simulink model "Lab05S"  (R2023b)
settings: Solver=VariableStepAuto  StartTime=0.0  StopTime=10.0  RelTol=1e-3
values from neighbouring files (symbols this model uses):
  A = [0 -1 5; 0 0 3; 0 0 -2]    [Lab01.m]    (also in Lab03.m = double(subs(A,x,x_eq)); Lab04.m = double(subs(A,[x u],[x_eq u_eq])); Lab05.m = [0 1; -3 -4])
  alpha = inv(-C*((A-B*K)\B))    [Lab04.m]    (also in Lab05.m; Prob1.m = 0.05; Prob2.m = 0.05; Prob3.m = 0.05)
  alpha_4 = inv(-C*((A-B*K_4)\B))    [Lab05.m]
  B = [1 1 1]'    [Lab01.m]    (also in Lab03.m = double(subs(B,u,u_eq)); Lab04.m = double(subs(B,[x u],[x_eq u_eq])); Lab05.m = [0 ; 1])
  B_reale = B.*epsilon    [Lab05.m]
  C = [0 0 5]    [Lab01.m]    (also in Lab03.m = double(subs(C,x,x_eq)); Lab04.m = double(subs(C,x,x_eq)); Lab05.m = [2 1])
  D = double(subs(D,u,u_eq))    [Lab03.m]    (also in Lab04.m; Lab05.m = 0)
  K = place(A,B,lambda_k)    [Lab04.m]    (also in Lab05.m)
  K_4 = place(A,B,lambda_k_4)    [Lab05.m]
  L = place(A',C',lambda_o)'    [Lab04.m]    (also in Lab05.m; Prob1.m = -Kc*Gp*Ga; Prob2.m = -Kc*Gp*Ga; Prob3.m = -Kc*Gp*Ga)
  L_6 = place(A',C',lambda_o_6)'    [Lab05.m]
  L_7 = place(A',C',lambda_o_7)'    [Lab05.m]
settings Model: Creator=matteo  LastModifiedBy=matteo

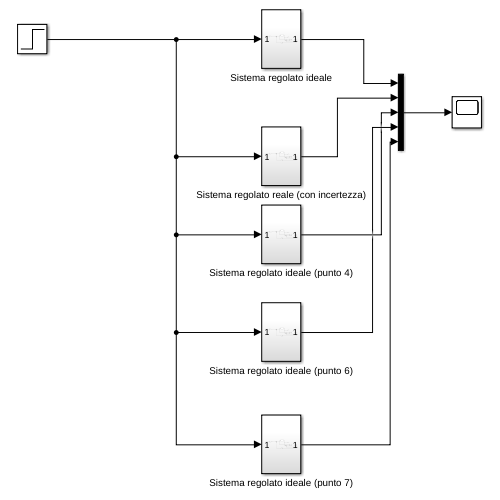
[thumbnail: Simulink's stored preview of the top-level diagram]
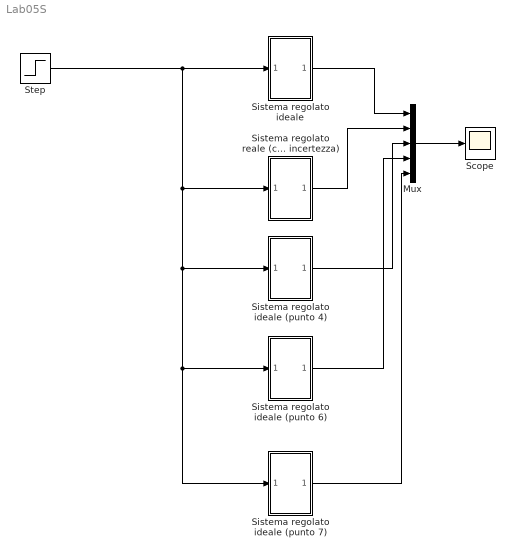
== system Lab05S ==
  Mux : Mux  Inputs=5
  Scope : Scope
  Sistema regolato ideale : Subsystem
  Sistema regolato ideale (punto 4) : Subsystem
  Sistema regolato ideale (punto 6) : Subsystem
  Sistema regolato ideale (punto 7) : Subsystem
  Sistema regolato reale (con incertezza) : Subsystem
  Step : Step  Time=0  SampleTime=0
  wires:
  Step/1 -> Sistema regolato ideale/1(In1), Sistema regolato reale (con incertezza)/1(In1), Sistema regolato ideale (punto 4)/1(In1), Sistema regolato ideale (punto 6)/1(In1), Sistema regolato ideale (punto 7)/1(In1)
  Sistema regolato ideale/1(Out1) -> Mux/1
  Mux/1 -> Scope/1
  Sistema regolato ideale (punto 4)/1(Out1) -> Mux/3
  Sistema regolato ideale (punto 6)/1(Out1) -> Mux/4
  Sistema regolato ideale (punto 7)/1(Out1) -> Mux/5
  Sistema regolato reale (con incertezza)/1(Out1) -> Mux/2

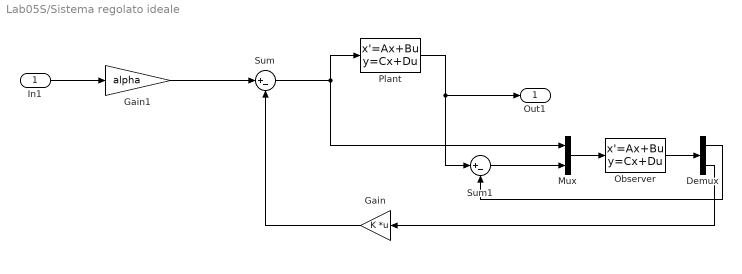
== system Lab05S/Sistema regolato ideale ==
  In1 : Inport
  Demux : Demux  Outputs=2
  Gain : Gain  Gain=K  Multiplication=Matrix(K*u)
  Gain1 : Gain  Gain=alpha
  Mux : Mux  Inputs=2
  Observer : StateSpace  A=A  B=[B L]  C=[C; eye(2)]  D=zeros(3,2)  InitialCondition=0
  Plant : StateSpace  A=A  B=B  C=C  D=D  InitialCondition=[0 0]'
  Sum : Sum  Inputs=|+-
  Sum1 : Sum  Inputs=|+-
  Out1 : Outport
  wires:
  Sum1/1 -> Mux/2
  In1/1 -> Gain1/1
  Gain/1 -> Sum/2
  Demux/1 -> Sum1/2
  Mux/1 -> Observer/1
  Observer/1 -> Demux/1
  Gain1/1 -> Sum/1
  Demux/2 -> Gain/1
  Sum/1 -> Mux/1, Plant/1
  Plant/1 -> Out1/1, Sum1/1

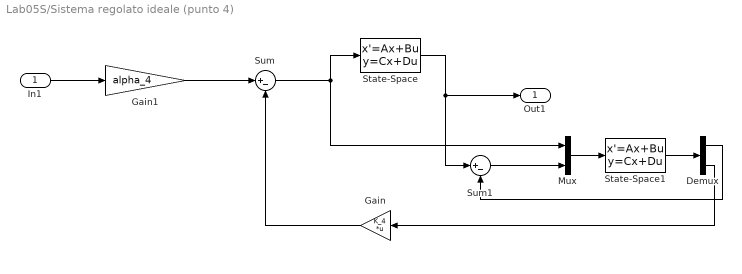
== system Lab05S/Sistema regolato ideale (punto 4) ==
  In1 : Inport
  Demux : Demux  Outputs=2
  Gain : Gain  Gain=K_4  Multiplication=Matrix(K*u)
  Gain1 : Gain  Gain=alpha_4
  Mux : Mux  Inputs=2
  State-Space : StateSpace  A=A  B=B  C=C  D=D  InitialCondition=[0 0]'
  State-Space1 : StateSpace  A=A  B=[B L]  C=[C; eye(2)]  D=zeros(3,2)  InitialCondition=0
  Sum : Sum  Inputs=|+-
  Sum1 : Sum  Inputs=|+-
  Out1 : Outport
  wires:
  Sum1/1 -> Mux/2
  In1/1 -> Gain1/1
  Gain/1 -> Sum/2
  Demux/1 -> Sum1/2
  Mux/1 -> State-Space1/1
  State-Space1/1 -> Demux/1
  Gain1/1 -> Sum/1
  Demux/2 -> Gain/1
  Sum/1 -> Mux/1, State-Space/1
  State-Space/1 -> Out1/1, Sum1/1

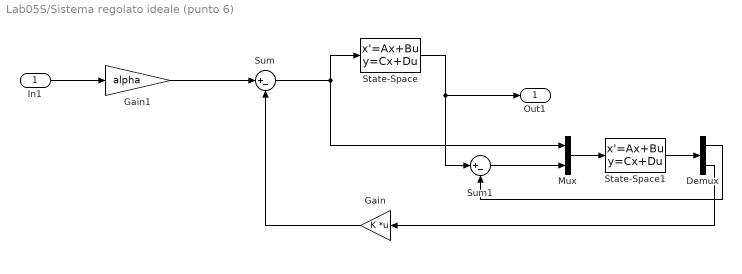
== system Lab05S/Sistema regolato ideale (punto 6) ==
  In1 : Inport
  Demux : Demux  Outputs=2
  Gain : Gain  Gain=K  Multiplication=Matrix(K*u)
  Gain1 : Gain  Gain=alpha
  Mux : Mux  Inputs=2
  State-Space : StateSpace  A=A  B=B  C=C  D=D  InitialCondition=[0 0]'
  State-Space1 : StateSpace  A=A  B=[B L_6]  C=[C; eye(2)]  D=zeros(3,2)  InitialCondition=0
  Sum : Sum  Inputs=|+-
  Sum1 : Sum  Inputs=|+-
  Out1 : Outport
  wires:
  Sum1/1 -> Mux/2
  In1/1 -> Gain1/1
  Gain/1 -> Sum/2
  Demux/1 -> Sum1/2
  Mux/1 -> State-Space1/1
  State-Space1/1 -> Demux/1
  Gain1/1 -> Sum/1
  Demux/2 -> Gain/1
  Sum/1 -> Mux/1, State-Space/1
  State-Space/1 -> Out1/1, Sum1/1

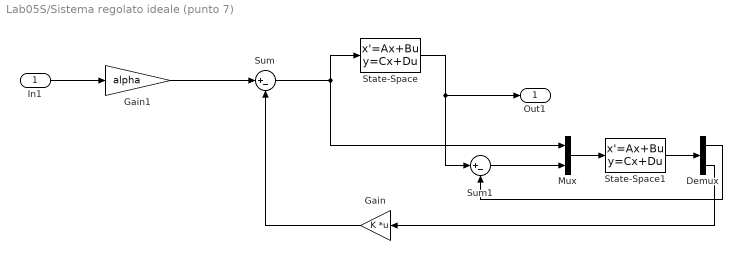
== system Lab05S/Sistema regolato ideale (punto 7) ==
  In1 : Inport
  Demux : Demux  Outputs=2
  Gain : Gain  Gain=K  Multiplication=Matrix(K*u)
  Gain1 : Gain  Gain=alpha
  Mux : Mux  Inputs=2
  State-Space : StateSpace  A=A  B=B  C=C  D=D  InitialCondition=[0 0]'
  State-Space1 : StateSpace  A=A  B=[B L_7]  C=[C; eye(2)]  D=zeros(3,2)  InitialCondition=0
  Sum : Sum  Inputs=|+-
  Sum1 : Sum  Inputs=|+-
  Out1 : Outport
  wires:
  Sum1/1 -> Mux/2
  In1/1 -> Gain1/1
  Gain/1 -> Sum/2
  Demux/1 -> Sum1/2
  Mux/1 -> State-Space1/1
  State-Space1/1 -> Demux/1
  Gain1/1 -> Sum/1
  Demux/2 -> Gain/1
  Sum/1 -> Mux/1, State-Space/1
  State-Space/1 -> Out1/1, Sum1/1

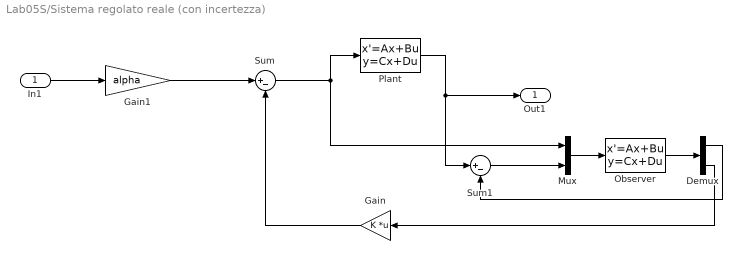
== system Lab05S/Sistema regolato reale (con incertezza) ==
  In1 : Inport
  Demux : Demux  Outputs=2
  Gain : Gain  Gain=K  Multiplication=Matrix(K*u)
  Gain1 : Gain  Gain=alpha
  Mux : Mux  Inputs=2
  Observer : StateSpace  A=A  B=[B L]  C=[C; eye(2)]  D=zeros(3,2)  InitialCondition=0
  Plant : StateSpace  A=A  B=B_reale  C=C  D=D  InitialCondition=[0 0]'
  Sum : Sum  Inputs=|+-
  Sum1 : Sum  Inputs=|+-
  Out1 : Outport
  wires:
  Sum1/1 -> Mux/2
  In1/1 -> Gain1/1
  Gain/1 -> Sum/2
  Demux/1 -> Sum1/2
  Mux/1 -> Observer/1
  Observer/1 -> Demux/1
  Gain1/1 -> Sum/1
  Demux/2 -> Gain/1
  Sum/1 -> Mux/1, Plant/1
  Plant/1 -> Out1/1, Sum1/1
